simulink model "rxnqca"  (R2020b)
settings: Solver=VariableStepAuto  StartTime=0.0  StopTime=0.1  RelTol=1e-3
settings Model: Creator=retou  LastModifiedBy=retou

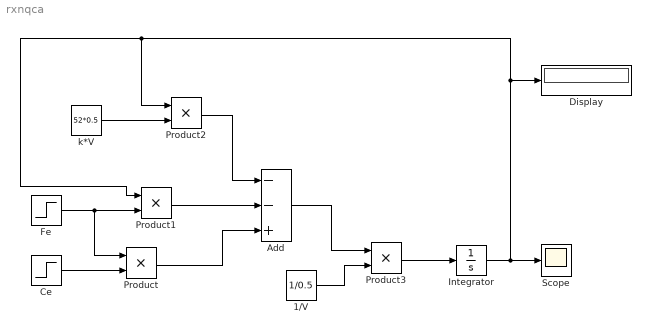
== system rxnqca ==
  1/V : Constant  Value=1/0.5
  Add : Sum  Inputs=--+
  Ce : Step  Time=0.05  Before=12  After=12*0.8  SampleTime=0
  Display : Display
  Fe : Step  Time=0  Before=100  After=100*1.2  SampleTime=0
  Integrator : Integrator  InitialCondition=9.523
  Product{,1..3} (4 alike) : Product
  Scope : Scope
  k*V : Constant  Value=52*0.5
  wires:
  Fe/1 -> Product1/2, Product/1
  Ce/1 -> Product/2
  k*V/1 -> Product2/2
  Integrator/1 -> Product2/1, Product1/1, Display/1, Scope/1
  Product/1 -> Add/3
  Product1/1 -> Add/2
  Product2/1 -> Add/1
  Add/1 -> Product3/1
  1/V/1 -> Product3/2
  Product3/1 -> Integrator/1
